simulink model "PubIfDecisionLSM_MDL"  (R2020b)
settings: configuration reference "DspaceConfig" (kept outside this file)
PostLoadFcn:
  | if any(exist('dsrtsu_mdlpostloadfcn', 'file') ~= 0), dsrtsu_mdlpostloadfcn('Execute', bdroot); end
InitFcn:
  | , if any(exist('rtifpga_mdlclblib', 'file') ~= 0), rtifpga_mdlclblib('Init', bdroot); end,
  | , if any(exist('dsmpb_private', 'file') ~= 0), dsmpb_private('dsmpb_mdlclblib', 'Init', bdroot); end,
values from neighbouring files (symbols this model uses):
  P_LSM_ALC_Enable = 0.0    [LSM_Parameter.sldd]
  P_LSM_AwayEdge_offset = 0.1    [LSM_Parameter.sldd]
  P_LSM_CentValidErr = 1.0    [LSM_Parameter.sldd]
  P_LSM_DOP_C0_EN_Limit = 0.8    [LSM_Parameter.sldd]
  P_LSM_DOP_C0_out_Limit = 2.0    [LSM_Parameter.sldd]
  P_LSM_DOP_C1_EN_Limit : value not decoded    [LSM_Parameter.sldd]
  P_LSM_DOP_C1_out_Limit : value not decoded    [LSM_Parameter.sldd]
  P_LSM_DOP_C1AndC2_Lim_X : value not decoded    [LSM_Parameter.sldd]
  P_LSM_DOP_C2_EN_Limit : value not decoded    [LSM_Parameter.sldd]
  P_LSM_DOP_C2_out_Limit : value not decoded    [LSM_Parameter.sldd]
  P_LSM_DOP_In_Pre2Dop_Dis = 1.0    [LSM_Parameter.sldd]
  P_LSM_DOP_Out_Pre2Dop_Dis = 2.0    [LSM_Parameter.sldd]
  P_LSM_DOP_PreDis_X : value not decoded    [LSM_Parameter.sldd]
  P_LSM_DOP_PreDis_Y : value not decoded    [LSM_Parameter.sldd]
  P_LSM_DOPEnableSW = 1.0    [LSM_Parameter.sldd]
  P_LSM_DOPValid_CheckTime = 0.06    [LSM_Parameter.sldd]
  P_LSM_DoubleLine_Curr2Cent_Dislimit = 0.5    [LSM_Parameter.sldd]
  P_LSM_DoubleLine_Dop2Cent_Dislimit = 0.5    [LSM_Parameter.sldd]
  P_LSM_DoubleLine_DOPOut_C1 : value not decoded    [LSM_Parameter.sldd]
  P_LSM_DoubleLine_Pre2Cent_Dislimit = 1.0    [LSM_Parameter.sldd]
  P_LSM_Error_Limit = 0.5    [LSM_Parameter.sldd]
  P_LSM_IFV2CenterAxis = 0.0    [LSM_Parameter.sldd]
  P_LSM_IFV2RearAxis = 0.0    [LSM_Parameter.sldd]
  P_LSM_Line2Edge_limit = 0.5    [LSM_Parameter.sldd]
  P_LSM_Line_Error = 0.1    [LSM_Parameter.sldd]
  P_LSM_LineSTD_Limit = 0.15    [LSM_Parameter.sldd]
  P_LSM_NOH_Switch = 0.0    [LSM_Parameter.sldd]
  P_LSM_OTL_C0_Factor = 1.0    [LSM_Parameter.sldd]
  P_LSM_OTL_C1_Factor = 0.5    [LSM_Parameter.sldd]
  P_LSM_OTL_C2_Factor = 0.5    [LSM_Parameter.sldd]
  P_LSM_Pre2OnlyLineDis = 5.0    [LSM_Parameter.sldd]
  P_LSM_Pre_t = 0.0    [LSM_Parameter.sldd]
  P_LSM_SingleLine_Cent2Edge_Dislimit = 100.0    [LSM_Parameter.sldd]
  P_LSM_SingleLine_Curr2Cent_Dislimit = 0.2    [LSM_Parameter.sldd]
  P_LSM_SingleLine_Dop2Cent_Dislimit = 0.2    [LSM_Parameter.sldd]
  P_LSM_SingleLine_DOPOut_C1 : value not decoded    [LSM_Parameter.sldd]
  P_LSM_SingleLine_Pre2Cent_Dislimit = 0.5    [LSM_Parameter.sldd]
  P_LSM_TJALimitSpd = 60.0    [LSM_Parameter.sldd]
undefined symbols (not defined in the file or in its folder): P_lCS_IFV2CenterAxis, P_LCS_IFV2RearAxis, P_LSM_EntryEdge_offset, P_LSM_EntryLnChngEnSwitch, P_LSM_EntryVanishDis, P_LSM_LinetLostTime, P_LSM_LineWijCal_C12, P_LSM_LineWijCal_C13, P_LSM_MapValid_ErrorSwitch, P_LSM_PosLineLcFac, P_LSM_SpdLim_Stub_Spd, P_LSM_SpdLim_StubLength, P_LSM_SpdTurnAlarm
libraries: simulink x324, TrueDurationTime x11
(part 13 of 25)

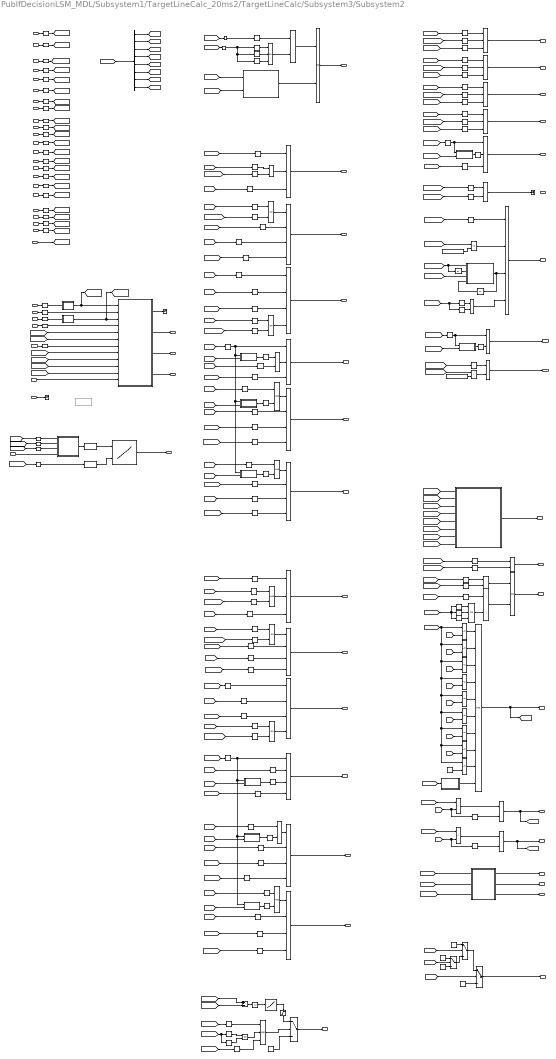
== system PubIfDecisionLSM_MDL/Subsystem1/TargetLineCalc_20ms2/TargetLineCalc/Subsystem3/Subsystem2 ==
  note: 推荐车道
  note: %%未走上汇出线,接管
  note: %%未走上汇出线,接管
  note: 高速或匝道汇出
  note: %%沿着汇出线驶出
  note: en_direction
      | 1 左驶出
      | 2 右驶出
      | 3 左直行
      | 4 右直行
      | 5 驶入
  note: %%未走上汇出线
  note: %%沿着汇出线驶出
  note: %%未走上汇出线
  note: 汇入
  note: 巡航（不存在有效路口）
  note: 左汇出
  note: 汇入或汇出路口有效
  note: 路口限速
  Exit_bIsLineExist : Inport
  f_distance : Inport  Port=2
  b_is_available : Inport  Port=3  OutDataTypeStr=uint8
  i_rec_lanes : Inport  Port=4
  nLaneID : Inport  Port=5
  en_direction : Inport  Port=6  OutDataTypeStr=uint8
  VehInRightmostLane : Inport  Port=7  OutDataTypeStr=boolean
  VehInLeftmostLane : Inport  Port=8  OutDataTypeStr=boolean
  nLaneNum : Inport  Port=9
  i_rec_lanes_num : Inport  Port=10
  " curr_b_vanish_valid" : Inport  Port=11
  " Exit_dDisStart" : Inport  Port=12
  Exit_dC0V : Inport  Port=13
  Entry_bIsLineExist : Inport  Port=14
  Entry_dDisStart : Inport  Port=15
  Entry_dC0V : Inport  Port=16
  " curr_f_vanish_pt_dis " : Inport  Port=17
  rightLane_valid : Inport  Port=18
  rightLane_type : Inport  Port=19
  leftLane_valid : Inport  Port=20
  leftLane_type : Inport  Port=21
  currentLane_type : Inport  Port=22
  VehSpd : Inport  Port=23
  f_end_dis : Inport  Port=24
  PilotRoadSts : Inport  Port=25
  left_b_vanish_valid : Inport  Port=26
  " left_f_vanish_pt_dis" : Inport  Port=27
  right_b_vanish_valid : Inport  Port=28
  right_f_vanish_pt_dis : Inport  Port=29
  currentLane_valid : Inport  Port=30
  HWASts : Inport  Port=31
  1-D Lookup Table : Lookup_n-D  NumberOfTableDimensions=1  BreakpointsForDimension1=P_LSM_SpdLim_StubLength  Table=P_LSM_SpdLim_Stub_Spd  TableDataTypeStr=uint8  ExtrapMethod=Clip  InternalRulePriority=Speed  OutDataTypeStr=uint8  RndMeth=Simplest  InputSameDT=on
  2-D Lookup Table : Lookup_n-D  BreakpointsForDimension1=[0,1,2,3,4,5]  BreakpointsForDimension2=P_LSM_SpdTurnAlarm  Table=reshape([0,1,1,1,1,1,0,0,1,1,1,1,0,0,0,1,1,1,0,0,0,0,1,1,0,0,0,0,0,1,0,0,0,0,0,1],6,6)  TableDataTypeStr=Inherit: Inherit from 'Table data'  InterpMethod=Nearest  InternalRulePriority=Speed  OutDataTypeStr=uint8  RndMeth=Simplest  InputSameDT=on
      settings: InputPortMap=u0,u1
  AND : Logic  AllPortsSameDT=off  OutDataTypeStr=boolean
  AND{1,3..5} (4 alike) : Logic  Operator=OR  AllPortsSameDT=off  OutDataTypeStr=boolean
  AND2 : Logic  AllPortsSameDT=off  OutDataTypeStr=boolean
  Abs : Abs
  Compare To Constant{1,4..5,12,75} (5 alike) : simulink/Logic and Bit Operations/Compare To Constant  relop=<  const=2  OutDataTypeStr=boolean
  Compare To Constant{10,16,46..47,56} (5 alike) : simulink/Logic and Bit Operations/Compare To Constant  relop===  const=5  OutDataTypeStr=boolean
  Compare To Constant11 : simulink/Logic and Bit Operations/Compare To Constant  relop===  const=3  OutDataTypeStr=boolean
  Compare To Constant{13,26,30,65,70,77} (6 alike) : simulink/Logic and Bit Operations/Compare To Constant  relop=<=  const=3  OutDataTypeStr=boolean
  Compare To Constant{14,28,45,48,50,52,61,83,85,95,97} (11 alike) : simulink/Logic and Bit Operations/Compare To Constant  relop===  const=0  OutDataTypeStr=boolean
  Compare To Constant{15,29,40,55,59,62,66,69,72,74,76,82,84,89,91,93} (16 alike) : simulink/Logic and Bit Operations/Compare To Constant  relop=>  const=0  OutDataTypeStr=boolean
  Compare To Constant{17,27,31,67} (4 alike) : simulink/Logic and Bit Operations/Compare To Constant  relop=<  const=1  OutDataTypeStr=boolean
  Compare To Constant{2,9,18..19,21,23..24,32,38,58,60,64,80,90} (14 alike) : simulink/Logic and Bit Operations/Compare To Constant  relop===  const=2  OutDataTypeStr=boolean
  Compare To Constant20 : simulink/Logic and Bit Operations/Compare To Constant  relop=~=  const=5  OutDataTypeStr=boolean
  Compare To Constant{7..8,22,33..35,37,39,51,68,71,81,88,96} (14 alike) : simulink/Logic and Bit Operations/Compare To Constant  relop===  const=1  OutDataTypeStr=boolean
  Compare To Constant25 : simulink/Logic and Bit Operations/Compare To Constant  relop=>  const=3  OutDataTypeStr=boolean
  Compare To Constant3 : simulink/Logic and Bit Operations/Compare To Constant  relop=~=  const=1  OutDataTypeStr=boolean
  Compare To Constant36 : simulink/Logic and Bit Operations/Compare To Constant  relop=~=  const=1  OutDataTypeStr=boolean
  Compare To Constant41 : simulink/Logic and Bit Operations/Compare To Constant  relop=>=  const=50  OutDataTypeStr=boolean
  Compare To Constant42 : simulink/Logic and Bit Operations/Compare To Constant  relop=~=  const=0  OutDataTypeStr=boolean
  Compare To Constant43 : simulink/Logic and Bit Operations/Compare To Constant  relop=~=  const=0  OutDataTypeStr=boolean
  Compare To Constant44 : simulink/Logic and Bit Operations/Compare To Constant  relop=>  const=50  OutDataTypeStr=boolean
  Compare To Constant49 : simulink/Logic and Bit Operations/Compare To Constant  relop===  const=4  OutDataTypeStr=boolean
  Compare To Constant53 : simulink/Logic and Bit Operations/Compare To Constant  relop=<=  const=50  OutDataTypeStr=boolean
  Compare To Constant54 : simulink/Logic and Bit Operations/Compare To Constant  relop=>  const=50  OutDataTypeStr=boolean
  Compare To Constant57 : simulink/Logic and Bit Operations/Compare To Constant  relop=<=  const=50  OutDataTypeStr=boolean
  Compare To Constant6 : simulink/Logic and Bit Operations/Compare To Constant  relop=>  const=3  OutDataTypeStr=boolean
  Compare To Constant63 : simulink/Logic and Bit Operations/Compare To Constant  relop=<  const=50  OutDataTypeStr=boolean
  Compare To Constant73 : simulink/Logic and Bit Operations/Compare To Constant  relop=<  const=50  OutDataTypeStr=boolean
  Compare To Constant78 : simulink/Logic and Bit Operations/Compare To Constant  relop=>=  const=50  OutDataTypeStr=boolean
  Compare To Constant79 : simulink/Logic and Bit Operations/Compare To Constant  relop=<  const=50  OutDataTypeStr=boolean
  Compare To Constant86 : simulink/Logic and Bit Operations/Compare To Constant  relop=>  const=1  OutDataTypeStr=boolean
  Compare To Constant87 : simulink/Logic and Bit Operations/Compare To Constant  relop=>  const=1  OutDataTypeStr=boolean
  Compare To Constant92 : simulink/Logic and Bit Operations/Compare To Constant  relop=~=  const=5  OutDataTypeStr=boolean
  Compare To Constant94 : simulink/Logic and Bit Operations/Compare To Constant  relop=~=  const=6  OutDataTypeStr=boolean
  Constant : Constant  Value=0  OutDataTypeStr=uint8
  Constant1 : Constant  OutDataTypeStr=uint8
  Constant2 : Constant  Value=2  OutDataTypeStr=uint8
  Constant3 : Constant  Value=0  OutDataTypeStr=uint8
  Constant4 : Constant  Value=0  OutDataTypeStr=uint8
  Constant5 : Constant  Value=60  OutDataTypeStr=uint8
  Constant6 : Constant  Value=P_LSM_EntryVanishDis
  Constant7 : Constant  Value=P_LSM_EntryVanishDis
  Data Type Conversion : DataTypeConversion
  Data Type Conversion1 : DataTypeConversion
  Demux : Demux  Outputs=8
  Logical Operator : Logic  Operator=OR  Inputs=3  AllPortsSameDT=off  OutDataTypeStr=boolean
  Logical Operator{1..2,4,8,17,21..22,24,28,31,33,35..37,39} (15 alike) : Logic  AllPortsSameDT=off  OutDataTypeStr=boolean
  Logical Operator{3,6,10,20,25..26,29..30} (8 alike) : Logic  Inputs=3  AllPortsSameDT=off  OutDataTypeStr=boolean
  Logical Operator11 : Logic  Inputs=10  AllPortsSameDT=off  OutDataTypeStr=boolean
  Logical Operator{5,12..13,15,18..19,23,32,34,40} (10 alike) : Logic  Inputs=4  AllPortsSameDT=off  OutDataTypeStr=boolean
  Logical Operator27 : Logic  Operator=OR  AllPortsSameDT=off  OutDataTypeStr=boolean
  Logical Operator38 : Logic  Operator=OR  AllPortsSameDT=off  OutDataTypeStr=boolean
  Logical Operator9 : Logic  Operator=OR  Inputs=3  AllPortsSameDT=off  OutDataTypeStr=boolean
  MATLAB Function : MATLAB Function  TreatAsAtomicUnit=on
  MATLAB Function1 : MATLAB Function  TreatAsAtomicUnit=on
  MATLAB Function2 : MATLAB Function  TreatAsAtomicUnit=on
  MATLAB Function3 : MATLAB Function  TreatAsAtomicUnit=on
  MATLAB Function4 : MATLAB Function  TreatAsAtomicUnit=on
  MATLAB Function5 : MATLAB Function  TreatAsAtomicUnit=on
  OR : Logic  Operator=OR  AllPortsSameDT=off  OutDataTypeStr=boolean
  OR1 : Logic  Inputs=3  AllPortsSameDT=off  OutDataTypeStr=boolean
  Relational Operator : RelationalOperator  Operator=>  OutDataTypeStr=boolean  RndMeth=Simplest
  Relational Operator1 : RelationalOperator  Operator=<=  OutDataTypeStr=boolean  RndMeth=Simplest
  Relational Operator{2..6,10,12..14} (9 alike) : RelationalOperator  Operator=~=  OutDataTypeStr=boolean  RndMeth=Simplest
  Relational Operator7 : RelationalOperator  Operator=>  OutDataTypeStr=boolean  RndMeth=Simplest
  Relational Operator8 : RelationalOperator  Operator=<  OutDataTypeStr=boolean  RndMeth=Simplest
  Saturation : Saturate  UpperLimit=60  LowerLimit=30  OutDataTypeStr=uint8
  Signal Copy{,1..32} (33 alike) : SignalConversion  OverrideOpt=off
  Subsystem : Subsystem
  Subsystem1 : Subsystem
  Subsystem10 : Subsystem
  Subsystem17 : Subsystem
  Subsystem19 : Subsystem
  Subsystem2 : Subsystem  Commented=on
  Subsystem3 : Subsystem
  Subsystem4 : Subsystem
  Subsystem5 : Subsystem
  Subsystem6 : Subsystem
  Subsystem8 : Subsystem
  Subsystem9 : Subsystem
  Subtract : Sum  Inputs=+-
  Switch{,1..3} (4 alike) : Switch  Criteria=u2 > Threshold
  Terminator : Terminator
  Terminator1 : Terminator
  Terminator4 : Terminator
  Unit Delay : UnitDelay  SampleTime=-1  HasFrameUpgradeWarning=on
  Unit Delay1 : UnitDelay  SampleTime=-1  HasFrameUpgradeWarning=on
  StubValid : Outport
  RightStub : Outport  Port=2
  LeftStub : Outport  Port=3
  CruiseValid : Outport  Port=4
  TurnLeft : Outport  Port=5
  TurnRight : Outport  Port=6
  rExitStub1 : Outport  Port=7
  rExitStub2 : Outport  Port=8
  rExitStub3 : Outport  Port=9
  Vanish_turnleft : Outport  Port=10
  EntryStub1 : Outport  Port=11
  CruiseRight : Outport  Port=12
  CruiseLeft : Outport  Port=13
  lExitStub1 : Outport  Port=14
  lExitStub2 : Outport  Port=15
  lExitStub3 : Outport  Port=16
  CruiseTurn : Outport  Port=17
  Forbid_TurnRight : Outport  Port=18
  Forbid_TurnLeft : Outport  Port=19
  OneLane : Outport  Port=20
  EntryStub2 : Outport  Port=21
  EntryStub3 : Outport  Port=22
  EntryStub4 : Outport  Port=23
  EntryStub5 : Outport  Port=24
  EntryStub6 : Outport  Port=25
  EntryStub5_TurnLeft : Outport  Port=26
  rExitStub4_takeover : Outport  Port=27
  lExitStub4_takeover : Outport  Port=28
  EntryStub5_takeover : Outport  Port=29
  Vanish_turnleft_takeover : Outport  Port=30
  turndir : Outport  Port=31
  roadClass : Outport  Port=32
  DecSpd : Outport  Port=33
  ForbidActive : Outport  Port=34
  StudLengthSpd : Outport  Port=35
  EntryStubVanishTurn : Outport  Port=36
  exitTakeOverValid : Outport  Port=37
  wires:
  [VehInLeftmostLane] -> Compare To Constant96/1
  Compare To Constant96/1 -> AND5/2
  Compare To Constant97/1 -> AND5/1
  [CruiseTurn] -> Compare To Constant97/1
  AND5/1 -> Logical Operator19/4
  Compare To Constant71/1 -> AND4/2
  [VehInRightmostLane] -> Compare To Constant71/1
  Compare To Constant95/1 -> AND4/1
  [CruiseTurn] -> Compare To Constant95/1
  AND4/1 -> Logical Operator15/4
  [f_vanish_pt_dis] -> MATLAB Function5/3(f_vanish_pt_dis)
  [b_vanish_valid] -> MATLAB Function5/1(b_vanish_valid), Unit Delay/1
  MATLAB Function5/1(VanishLaneTkOverValid) -> Logical Operator40/3, Unit Delay1/1
  Unit Delay1/1 -> MATLAB Function5/4(VanishLaneTkOverValidK)
  Unit Delay/1 -> MATLAB Function5/2(b_vanish_validK)
  Constant7/1 -> Relational Operator1/2
  Logical Operator4/1 -> Logical Operator40/4  "EntryStub5_takeover"
  Compare To Constant94/1 -> Logical Operator4/2
  Compare To Constant92/1 -> Logical Operator4/1
  [HWASts] -> Compare To Constant92/1, Compare To Constant94/1
  HWASts/1 -> [HWASts]
  Constant6/1 -> Relational Operator/2
  Logical Operator2/1 -> EntryStubVanishTurn/1  "EntryStub5_takeover"
  [f_vanish_pt_dis] -> Relational Operator/1
  Relational Operator/1 -> Logical Operator2/2
  [b_vanish_valid] -> Compare To Constant93/1
  Compare To Constant93/1 -> Logical Operator2/1
  Saturation/1 -> Switch3/1
  Compare To Constant91/1 -> OR1/3
  [f_distance] -> Compare To Constant91/1
  Switch3/1 -> StudLengthSpd/1
  Constant5/1 -> Switch3/3
  1-D Lookup Table/1 -> Saturation/1
  Abs/1 -> 1-D Lookup Table/1
  Subtract/1 -> Abs/1
  OR1/1 -> Switch3/2
  [f_end_dis] -> Subtract/1
  [f_distance] -> Subtract/2
  OR/1 -> OR1/2
  Compare To Constant89/1 -> OR1/1
  Compare To Constant90/1 -> OR/2
  Compare To Constant88/1 -> OR/1
  [b_is_available] -> Compare To Constant89/1
  [en_direction] -> Compare To Constant88/1, Compare To Constant90/1
  Compare To Constant87/1 -> Logical Operator5/4
  [f_distance] -> Compare To Constant87/1
  Compare To Constant86/1 -> Logical Operator12/4
  [f_distance] -> Compare To Constant86/1
  MATLAB Function1/4(ForbidActive) -> ForbidActive/1
  currentLane_valid/1 -> MATLAB Function1/12(currentLane_valid)
  MATLAB Function1/3(DecSpd) -> DecSpd/1
  AND3/1 -> Logical Operator5/1
  [CruiseTurn] -> Compare To Constant85/1
  Compare To Constant85/1 -> AND3/1
  AND2/1 -> Logical Operator20/2
  Compare To Constant84/1 -> AND2/1
  [CruiseTurn] -> Compare To Constant84/1
  AND1/1 -> Logical Operator12/1
  [CruiseTurn] -> Compare To Constant83/1
  Compare To Constant83/1 -> AND1/1
  AND/1 -> Logical Operator3/2
  Compare To Constant82/1 -> AND/1
  [CruiseTurn] -> Compare To Constant82/1
  Data Type Conversion1/1 -> 2-D Lookup Table/2
  Data Type Conversion/1 -> 2-D Lookup Table/1
  2-D Lookup Table/1 -> exitTakeOverValid/1
  MATLAB Function2/1(y) -> Data Type Conversion/1
  [en_direction] -> Signal Copy26/1
  [nLaneID] -> Signal Copy25/1
  [bit1] -> Signal Copy24/1
  [f_distance] -> Signal Copy27/1
  [dDisStart] -> Compare To Constant13/1
  Compare To Constant13/1 -> Logical Operator22/1
  Logical Operator1/1 -> Logical Operator6/2  "rExitStub2"
  [dDisStart] -> Compare To Constant26/1
  Compare To Constant26/1 -> Logical Operator1/2
  MATLAB Function1/2(roadClass) -> roadClass/1
  Signal Copy23/1 -> MATLAB Function1/7(currentLane_type)
  currentLane_type/1 -> Signal Copy23/1
  Signal Copy22/1 -> MATLAB Function1/4(leftLane_type)
  Signal Copy21/1 -> MATLAB Function1/2(rightLane_type)
  leftLane_type/1 -> Signal Copy22/1
  rightLane_type/1 -> Signal Copy21/1
  MATLAB Function1/1(turndir) -> Terminator/1
  Signal Copy20/1 -> Subsystem1/1(In1)
  Signal Copy19/1 -> Subsystem/1(In1)
  [b_vanish_valid] -> MATLAB Function1/5(curr_vanish_valid)
  leftLane_valid/1 -> Signal Copy20/1
  rightLane_valid/1 -> Signal Copy19/1
  Signal Copy2/1 -> [Entry_dDisStart]
  Signal Copy18/1 -> [Entry_dC0V]
  Signal Copy17/1 -> [Entry_bIsLineExist]
  Signal Copy16/1 -> [dDisStart]
  Signal Copy15/1 -> [dC0V]
  Signal Copy14/1 -> [bIsLineExist]
  Signal Copy13/1 -> [en_direction]
  Signal Copy12/1 -> [f_distance]
  Signal Copy11/1 -> [b_is_available]
  Signal Copy10/1 -> [f_vanish_pt_dis]
  Signal Copy9/1 -> [b_vanish_valid]
  Signal Copy8/1 -> [i_rec_lanes_num]
  Signal Copy7/1 -> [nLaneNum]
  Signal Copy6/1 -> [VehInLeftmostLane]
  Signal Copy5/1 -> [VehInRightmostLane]
  Signal Copy4/1 -> [nLaneID]
  Signal Copy3/1 -> [i_rec_lanes]
  Logical Operator/1 -> Logical Operator28/2
  Compare To Constant49/1 -> Logical Operator/3
  Compare To Constant50/1 -> Logical Operator/1
  Compare To Constant11/1 -> Logical Operator/2
  Signal Copy1/1 -> Compare To Constant8/1, Compare To Constant9/1, Compare To Constant10/1  "LSM_en_direction_stub"
  Signal Copy/1 -> Compare To Constant7/1  "LSM_B_IS_Available"
  [bIsLineExist] -> Compare To Constant32/1
  Logical Operator40/1 -> EntryStub5_takeover/1  "EntryStub5_takeover"
  Compare To Constant76/1 -> Logical Operator40/1
  [b_vanish_valid] -> Compare To Constant76/1
  Compare To Constant75/1 -> Logical Operator39/2
  Logical Operator39/1 -> Logical Operator27/1
  [Entry_bIsLineExist] -> Compare To Constant75/1
  Logical Operator38/1 -> StubValid/1  "StubValid"
  Subsystem17/1(enStubExist) -> Logical Operator38/2
  [Entry_bIsLineExist] -> Subsystem17/2(Entry_bIsLineExist)
  [b_is_available] -> Subsystem17/1(b_is_available)
  Logical Operator37/1 -> Vanish_turnleft_takeover/1  "Vanish_turnleft_takeover"
  Compare To Constant74/1 -> Logical Operator37/1  "Vanish_turnleft"
  [b_vanish_valid] -> Compare To Constant74/1
  Compare To Constant73/1 -> Logical Operator37/2  "Vanish_turnleft_takeover"
  [f_vanish_pt_dis] -> Compare To Constant73/1
  Logical Operator36/1 -> Terminator1/1  "EntryStub5_TurnLeft"
  Compare To Constant72/1 -> Logical Operator36/2
  [f_vanish_pt_dis] -> Compare To Constant72/1
  " curr_f_vanish_pt_dis "/1 -> Signal Copy10/1
  Relational Operator1/1 -> Logical Operator40/2
  [f_vanish_pt_dis] -> Relational Operator1/1
  Compare To Constant69/1 -> Logical Operator35/2
  Compare To Constant70/1 -> Logical Operator35/1
  [dDisStart] -> Compare To Constant70/1
  [dC0V] -> Subsystem5/2(u)
  Subsystem5/1(y) -> Compare To Constant69/1
  Compare To Constant68/1 -> Logical Operator34/3
  [en_direction] -> Compare To Constant68/1
  [f_distance] -> Compare To Constant67/1
  Logical Operator34/1 -> lExitStub4_takeover/1  "lExitStub4_takeover"
  Logical Operator35/1 -> Logical Operator34/1
  Compare To Constant67/1 -> Logical Operator34/2
  Subsystem10/1(y) -> Compare To Constant66/1
  [dC0V] -> Subsystem10/2(u)
  [dDisStart] -> Compare To Constant65/1
  Compare To Constant65/1 -> Logical Operator33/1
  Compare To Constant66/1 -> Logical Operator33/2
  Logical Operator33/1 -> Logical Operator32/1
  Logical Operator32/1 -> rExitStub4_takeover/1  "rExitStub4_takeover"
  [f_end_dis] -> Compare To Constant63/1
  [en_direction] -> Compare To Constant64/1
  Compare To Constant64/1 -> Logical Operator32/2
  [b_vanish_valid] -> Compare To Constant62/1
  Compare To Constant62/1 -> Logical Operator36/1
  [Entry_bIsLineExist] -> Compare To Constant60/1
  Compare To Constant60/1 -> Logical Operator31/1, Subsystem8/1(laneValid)
  [Entry_dC0V] -> Subsystem8/2(u)
  Subsystem8/1(y) -> Compare To Constant61/1
  Compare To Constant61/1 -> Logical Operator31/2
  Logical Operator31/1 -> EntryStub6/1  "EntryStub6"
  Logical Operator30/1 -> EntryStub5/1  "EntryStub5"
  Compare To Constant59/1 -> Logical Operator30/2
  Subsystem6/1(y) -> Compare To Constant59/1
  [Entry_dC0V] -> Subsystem6/2(u)
  Compare To Constant58/1 -> Logical Operator30/1, Subsystem6/1(laneValid)
  [Entry_bIsLineExist] -> Compare To Constant58/1
  Logical Operator25/1 -> EntryStub3/1  "EntryStub3"
  [en_direction] -> Compare To Constant47/1  "LSM_Stub_Direction"
  [b_vanish_valid] -> Compare To Constant15/1
  Compare To Constant15/1 -> Logical Operator25/2
  Compare To Constant47/1 -> Logical Operator25/1
  [f_distance] -> Compare To Constant54/1
  Compare To Constant54/1 -> Logical Operator25/3
  Compare To Constant57/1 -> Logical Operator29/3
  [f_distance] -> Compare To Constant57/1
  Compare To Constant56/1 -> Logical Operator29/1
  Compare To Constant55/1 -> Logical Operator29/2
  [b_vanish_valid] -> Compare To Constant55/1
  [en_direction] -> Compare To Constant56/1  "LSM_Stub_Direction"
  Logical Operator29/1 -> EntryStub4/1  "EntryStub4"
  Logical Operator26/1 -> EntryStub2/1  "EntryStub2"
  [en_direction] -> Compare To Constant46/1  "LSM_Stub_Direction"
  [b_vanish_valid] -> Compare To Constant45/1
  Compare To Constant45/1 -> Logical Operator26/2
  Compare To Constant46/1 -> Logical Operator26/1
  [f_distance] -> Compare To Constant53/1
  Compare To Constant53/1 -> Logical Operator26/3
  Compare To Constant44/1 -> Logical Operator10/3
  [f_distance] -> Compare To Constant44/1
  Entry_bIsLineExist/1 -> Signal Copy17/1
  Entry_dDisStart/1 -> Signal Copy2/1
  Entry_dC0V/1 -> Signal Copy18/1
  i_rec_lanes/1 -> Signal Copy3/1
  Demux/2 -> [bit2]
  Demux/3 -> [bit3]
  Demux/1 -> [bit1]
  Demux/8 -> [bit8]
  Demux/7 -> [bit7]
  Demux/6 -> [bit6]
  Demux/4 -> [bit4]
  Demux/5 -> [bit5]
  [i_rec_lanes] -> Demux/1
  Logical Operator24/1 -> [TurnRight], TurnRight/1  "TurnRight"
  Compare To Constant43/1 -> Logical Operator24/2
  Logical Operator21/1 -> [TurnLeft], TurnLeft/1  "TurnLeft"
  Compare To Constant42/1 -> Logical Operator21/2
  Compare To Constant21/1 -> Logical Operator13/3
  Compare To Constant3/1 -> AND/2
  [nLaneID] -> Relational Operator7/1
  Relational Operator5/1 -> Logical Operator11/4
  Relational Operator3/1 -> Logical Operator11/2
  Logical Operator15/1 -> rExitStub1/1  "rExitStub1"
  [en_direction] -> Compare To Constant21/1
  Compare To Constant24/1 -> Logical Operator15/3
  en_direction/1 -> Signal Copy13/1
  [nLaneID] -> Relational Operator3/1, Relational Operator4/1, Relational Operator5/1, Relational Operator10/1, Relational Operator12/1, Relational Operator14/1, Relational Operator13/1, Relational Operator6/1, Relational Operator2/1
  Relational Operator6/1 -> Logical Operator11/5
  [f_distance] -> Compare To Constant17/1
  Compare To Constant16/1 -> Logical Operator10/1
  Compare To Constant2/1 -> Logical Operator3/1
  [bit4] -> Relational Operator5/2
  [en_direction] -> Compare To Constant24/1
  " curr_b_vanish_valid"/1 -> Signal Copy9/1
  Logical Operator13/1 -> rExitStub3/1  "rExitStub3"
  Compare To Constant7/1 -> Logical Operator8/1
  [VehInRightmostLane] -> Compare To Constant3/1
  Exit_dC0V/1 -> Signal Copy15/1
  [bit5] -> Relational Operator6/2
  Compare To Constant14/1 -> Logical Operator10/2
  [bit3] -> Relational Operator4/2
  [bit2] -> Relational Operator3/2
  Compare To Constant25/1 -> Logical Operator15/2
  Logical Operator3/1 -> RightStub/1  "RightStub"
  [dDisStart] -> Compare To Constant25/1
  [b_vanish_valid] -> Compare To Constant14/1
  i_rec_lanes_num/1 -> Signal Copy8/1
  nLaneNum/1 -> Signal Copy7/1
  Logical Operator17/1 -> Logical Operator13/1
  [en_direction] -> Compare To Constant16/1  "LSM_Stub_Direction"
  [bit1] -> Relational Operator7/2, Compare To Constant42/1
  Relational Operator8/1 -> Logical Operator24/1
  [nLaneID] -> Relational Operator8/1
  [bit1] -> Relational Operator8/2, Compare To Constant43/1
  [bit1] -> Relational Operator2/2
  Relational Operator4/1 -> Logical Operator11/3
  Relational Operator2/1 -> Logical Operator11/1
  [en_direction] -> Compare To Constant2/1  "LSM_Stub_Direction"
  f_distance/1 -> Signal Copy12/1
  VehInLeftmostLane/1 -> Signal Copy6/1
  nLaneID/1 -> Signal Copy4/1
  " Exit_dDisStart"/1 -> Signal Copy16/1
  VehInRightmostLane/1 -> Signal Copy5/1
  Compare To Constant17/1 -> Logical Operator13/2
  Logical Operator11/1 -> [CruiseTurn], CruiseTurn/1  "CruiseTurn"
  Logical Operator10/1 -> EntryStub1/1  "EntryStub1"
  [VehInRightmostLane] -> Compare To Constant22/1
  Logical Operator12/1 -> CruiseRight/1  "CruiseRight"
  Compare To Constant22/1 -> AND1/2
  Compare To Constant19/1 -> Logical Operator12/2
  [en_direction] -> Compare To Constant19/1  "LSM_Stub_Direction"
  b_is_available/1 -> Signal Copy11/1
  [b_is_available] -> Signal Copy/1
  [bIsLineExist] -> Compare To Constant1/1
  Compare To Constant1/1 -> Logical Operator3/3
  Exit_bIsLineExist/1 -> Signal Copy14/1
  [bIsLineExist] -> Compare To Constant12/1
  [bIsLineExist] -> Compare To Constant18/1
  Compare To Constant18/1 -> Logical Operator15/1
  Compare To Constant23/1 -> Logical Operator6/1, Subsystem19/1(laneValid), Subsystem9/1(laneValid), Subsystem10/1(laneValid)
  [bIsLineExist] -> Compare To Constant23/1
  Logical Operator6/1 -> rExitStub2/1  "rExitStub2"
  [bIsLineExist] -> Compare To Constant4/1
  Compare To Constant4/1 -> Logical Operator20/3
  [bIsLineExist] -> Compare To Constant5/1
  Compare To Constant36/1 -> AND2/2
  Compare To Constant5/1 -> Logical Operator5/3
  Compare To Constant34/1 -> Logical Operator20/1
  [en_direction] -> Compare To Constant34/1  "LSM_Stub_Direction"
  Compare To Constant33/1 -> Logical Operator5/2
  Compare To Constant35/1 -> AND3/2
  [VehInLeftmostLane] -> Compare To Constant35/1
  [VehInLeftmostLane] -> Compare To Constant36/1
  Logical Operator5/1 -> CruiseLeft/1  "CruiseLeft"
  [en_direction] -> Compare To Constant33/1  "LSM_Stub_Direction"
  Logical Operator20/1 -> LeftStub/1  "LeftStub"
  Logical Operator23/1 -> lExitStub2/1  "lExitStub2"
  [bIsLineExist] -> Compare To Constant38/1
  Compare To Constant38/1 -> Subsystem3/1(laneValid), Subsystem5/1(laneValid), Subsystem4/1(laneValid), Logical Operator23/1
  Compare To Constant32/1 -> Logical Operator19/1
  Compare To Constant31/1 -> Logical Operator18/2
  Logical Operator22/1 -> Logical Operator18/1
  Logical Operator18/1 -> lExitStub3/1  "lExitStub3"
  [en_direction] -> Compare To Constant39/1
  [f_distance] -> Compare To Constant31/1
  Compare To Constant39/1 -> Logical Operator19/3
  [en_direction] -> Compare To Constant37/1
  Logical Operator19/1 -> lExitStub1/1  "lExitStub1"
  Compare To Constant37/1 -> Logical Operator18/3
  Compare To Constant48/1 -> Logical Operator39/1
  [b_is_available] -> Compare To Constant48/1
  Relational Operator10/1 -> Logical Operator11/6
  Relational Operator12/1 -> Logical Operator11/7
  Relational Operator13/1 -> Logical Operator11/8
  [bit6] -> Relational Operator10/2
  [bit7] -> Relational Operator12/2
  [bit8] -> Relational Operator13/2
  Relational Operator7/1 -> Logical Operator21/1
  [en_direction] -> Signal Copy1/1
  Compare To Constant8/1 -> Logical Operator9/1
  Compare To Constant9/1 -> Logical Operator9/2
  Compare To Constant10/1 -> Logical Operator9/3
  Logical Operator9/1 -> Logical Operator8/2
  Logical Operator8/1 -> Logical Operator38/1  "LSM_B_StubValid"
  Compare To Constant12/1 -> Logical Operator12/3
  Relational Operator14/1 -> Logical Operator11/9
  Constant/1 -> Relational Operator14/2
  Logical Operator28/1 -> Logical Operator27/2
  [en_direction] -> Compare To Constant49/1, Compare To Constant11/1, Compare To Constant50/1
  [b_is_available] -> Compare To Constant51/1
  Compare To Constant51/1 -> Logical Operator28/1
  Logical Operator27/1 -> CruiseValid/1  "CruiseValid"
  [i_rec_lanes] -> MATLAB Function/2(i_rec_lanes)
  [nLaneID] -> MATLAB Function/1(nLaneID)
  MATLAB Function/1(Forbid_TurnRight) -> Forbid_TurnRight/1
  MATLAB Function/2(Forbid_TurnLeft) -> Forbid_TurnLeft/1
  MATLAB Function/3(OneLane) -> OneLane/1
  [i_rec_lanes_num] -> MATLAB Function/3(i_rec_lanes_num)
  Subsystem19/1(y) -> Compare To Constant52/1
  [dC0V] -> Subsystem19/2(u)
  Compare To Constant52/1 -> Logical Operator1/1
  Compare To Constant29/1 -> Logical Operator17/2
  Compare To Constant77/1 -> Logical Operator17/1
  [dDisStart] -> Compare To Constant77/1
  [dC0V] -> Subsystem9/2(u)
  Subsystem9/1(y) -> Compare To Constant29/1
  [dDisStart] -> Compare To Constant6/1
  Compare To Constant6/1 -> Logical Operator19/2
  Compare To Constant28/1 -> Logical Operator23/3
  Compare To Constant30/1 -> Logical Operator23/2
  [dDisStart] -> Compare To Constant30/1
  [dC0V] -> Subsystem4/2(u)
  Subsystem4/1(y) -> Compare To Constant28/1
  Subsystem3/1(y) -> Compare To Constant40/1
  [dC0V] -> Subsystem3/2(u)
  Compare To Constant40/1 -> Logical Operator22/2
  [i_rec_lanes] -> MATLAB Function3/1(i_rec_lanes)
  MATLAB Function3/1(y) -> Logical Operator11/10
  Signal Copy24/1 -> MATLAB Function2/1(nLaneNum)  "LSM_nLaneNum"
  Signal Copy25/1 -> MATLAB Function2/2(nLaneID)  "LSM_nLaneID"
  Signal Copy26/1 -> MATLAB Function2/3(en_direction)
  Signal Copy27/1 -> Data Type Conversion1/1  "LSM_f_distance"
  f_end_dis/1 -> Signal Copy28/1
  Signal Copy28/1 -> [f_end_dis]
  [f_distance] -> Compare To Constant27/1
  Compare To Constant27/1 -> Logical Operator32/3
  [f_end_dis] -> Compare To Constant41/1
  Compare To Constant41/1 -> Logical Operator13/4
  [f_end_dis] -> Compare To Constant78/1
  Compare To Constant78/1 -> Logical Operator18/4
  [f_end_dis] -> Compare To Constant79/1
  Compare To Constant79/1 -> Logical Operator34/4
  Subsystem/1(y) -> MATLAB Function1/1(rightLane_valid), [rightLane_valid]
  Subsystem1/1(y) -> MATLAB Function1/3(leftLane_valid), [leftLane_valid]
  VehSpd/1 -> Terminator4/1
  PilotRoadSts/1 -> MATLAB Function2/4(PilotRoadSts)
  left_b_vanish_valid/1 -> Signal Copy30/1
  " left_f_vanish_pt_dis"/1 -> Signal Copy29/1
  Signal Copy30/1 -> [left_b_vanish_valid]
  Signal Copy29/1 -> [left_f_vanish_pt_dis]
  Signal Copy31/1 -> [right_f_vanish_pt_dis]
  Signal Copy32/1 -> [right_b_vanish_valid]
  right_f_vanish_pt_dis/1 -> Signal Copy31/1
  right_b_vanish_valid/1 -> Signal Copy32/1
  [f_vanish_pt_dis] -> MATLAB Function1/6(curr_vanish_pt_dis)
  [left_b_vanish_valid] -> MATLAB Function1/8(left_vanish_valid)
  [left_f_vanish_pt_dis] -> MATLAB Function1/9(left_vanish_pt_dis)
  [right_b_vanish_valid] -> MATLAB Function1/10(right_vanish_valid)
  [right_f_vanish_pt_dis] -> MATLAB Function1/11(right_vanish_pt_dis)
  MATLAB Function4/1(y) -> Vanish_turnleft/1
  [b_vanish_valid] -> MATLAB Function4/3(curr_vanish_valid)
  [f_vanish_pt_dis] -> MATLAB Function4/4(curr_vanish_pt_dis)
  [right_f_vanish_pt_dis] -> MATLAB Function4/8(right_vanish_pt_dis)
  [right_b_vanish_valid] -> MATLAB Function4/7(right_vanish_valid)
  [left_f_vanish_pt_dis] -> MATLAB Function4/6(left_vanish_pt_dis)
  [left_b_vanish_valid] -> MATLAB Function4/5(left_vanish_valid)
  [leftLane_valid] -> MATLAB Function4/2(leftLane_valid)
  [rightLane_valid] -> MATLAB Function4/1(rightLane_valid)
  Compare To Constant63/1 -> Logical Operator32/4
  [CruiseTurn] -> Switch/2
  Switch/1 -> turndir/1
  [TurnLeft] -> Switch1/2
  Constant1/1 -> Switch1/1
  [TurnRight] -> Switch2/2
  Constant2/1 -> Switch2/1
  Switch2/1 -> Switch1/3
  Switch1/1 -> Switch/1
  Constant3/1 -> Switch2/3
  Constant4/1 -> Switch/3
  Compare To Constant20/1 -> Logical Operator30/3
  [en_direction] -> Compare To Constant20/1  "LSM_Stub_Direction"
  [en_direction] -> Compare To Constant80/1
  Compare To Constant80/1 -> Logical Operator6/3
  Compare To Constant81/1 -> Logical Operator23/4
  [en_direction] -> Compare To Constant81/1

== system PubIfDecisionLSM_MDL/Subsystem1/TargetLineCalc_20ms2/TargetLineCalc/Subsystem3/Subsystem3 ==
  PilotTurnSwSts : Inport
  nLaneID : Inport  Port=2
  Compare To Constant2 : simulink/Logic and Bit Operations/Compare To Constant  relop===  const=1  OutDataTypeStr=boolean
  Compare To Constant3 : simulink/Logic and Bit Operations/Compare To Constant  relop===  const=2  OutDataTypeStr=boolean
  Constant : Constant  OutDataTypeStr=uint8
  Constant1 : Constant  Value=2  OutDataTypeStr=uint8
  Constant2 : Constant  Value=0  OutDataTypeStr=uint8
  Logical Operator1 : Logic  AllPortsSameDT=off  OutDataTypeStr=boolean
  Logical Operator2 : Logic  AllPortsSameDT=off  OutDataTypeStr=boolean
  Relational Operator1 : RelationalOperator  Operator=<  OutDataTypeStr=boolean  RndMeth=Simplest
  Relational Operator2 : RelationalOperator  Operator=>  OutDataTypeStr=boolean  RndMeth=Simplest
  Switch : Switch  Criteria=u2 > Threshold
  Switch1 : Switch  Criteria=u2 > Threshold
  Unit Delay{,1..3} (4 alike) : UnitDelay  SampleTime=-1  HasFrameUpgradeWarning=on
  LaneChange : Outport
  wires:
  Switch/1 -> LaneChange/1  "LaneChange"
  Relational Operator2/1 -> Logical Operator2/2
  nLaneID/1 -> Relational Operator1/1, Unit Delay/1, Unit Delay1/1, Relational Operator2/1
  Switch1/1 -> Switch/3
  Compare To Constant3/1 -> Logical Operator2/1
  Unit Delay1/1 -> Relational Operator2/2
  Constant1/1 -> Switch1/1
  Unit Delay3/1 -> Compare To Constant2/1
  Logical Operator2/1 -> Switch1/2
  PilotTurnSwSts/1 -> Unit Delay3/1, Unit Delay2/1
  Unit Delay/1 -> Relational Operator1/2
  Logical Operator1/1 -> Switch/2
  Unit Delay2/1 -> Compare To Constant3/1
  Constant2/1 -> Switch1/3
  Constant/1 -> Switch/1
  Compare To Constant2/1 -> Logical Operator1/1
  Relational Operator1/1 -> Logical Operator1/2

== system PubIfDecisionLSM_MDL/Subsystem1/TargetLineCalc_20ms2/TargetLineCalc/Subsystem3/Subsystem4 ==
  PilotRoadSts : Inport
  en_direction : Inport  Port=2
  f_vanish_pt_dis : Inport  Port=3
  changeVoice : Inport  Port=4
  b_vanish_valid : Inport  Port=5
  exitTakeOverValid : Inport  Port=6
  lExitStub4_takeover : Inport  Port=7
  rExitStub4_takeover : Inport  Port=8
  f_distance : Inport  Port=9
  Double_Line_Lost : Inport  Port=10
  LaneNum : Inport  Port=11
  NoPUCR : Inport  Port=12
  NoPUCR_Dis : Inport  Port=13
  HWASts : Inport  Port=14
  Chart : Stateflow chart  TreatAsAtomicUnit=on
      settings: PortSchema="{\"entries\":[{\"content\":{\"sides\":[{\"content\":{\"connectorIds\":[\"In1\",\"In7\",\"In2\",\"In3\",\"In4\",\"In5\",\"In6\",\"In8\",\"In9\",\"In10\",\"In11\",\"In12\",\"In13\",\"In14\",\"In15\"]},\"type\":\"ConnectorPlacement.EquallySpacedRectSide\",\"uuid\":\"ffbd8463-567a-4659-b8b5-1d92828b502e\"},{\"content\":{\"connectorIds\":[\"Out1\"],\"side\":\"RIGHT\"},\"type\":\"ConnectorPlacement.EquallySpacedRectSide\",\"uuid\":\"a8d4ede4-058c-411e-a1bb-a05fa58933cd\"},{\"content\":{\"connectorIds\":[],\"side\":\"TOP\"},\"type\":\"ConnectorPlacement.EquallySpacedRectSide\",\"uuid\":\"cb34091e-f6c1-4e39-8b68-2bb4c65a08b7\"},{\"content\":{\"connectorIds\":[],\"side\":\"HIDDEN\"},\"type\":\"ConnectorPlacement.EquallySpacedRectSide\",\"uuid\":\"3139b7f1-1c79-4b06-a78a-de5284464f98\"}]},\"type\":\"ConnectorPlacement.EquallySpacedConnector\",\"uuid\":\"8437a6c5-b71e-48c0-980a-51389f42da06\"}],\"packageUris\":[\"http://schema.mathworks.com/mf0/Connector/R2020b\"],\"version\":\"1.0\"}"
  Compare To Constant1 : simulink/Logic and Bit Operations/Compare To Constant  relop=>  const=0  OutDataTypeStr=boolean
  Compare To Constant67 : simulink/Logic and Bit Operations/Compare To Constant  relop=>  const=0  OutDataTypeStr=boolean
  Constant : Constant  Value=P_LSM_EntryVanishDis
  OR : Logic  Operator=OR  AllPortsSameDT=off  OutDataTypeStr=boolean
  Signal Copy{5..6,8,10..12} (6 alike) : SignalConversion  OverrideOpt=off
  Unit Delay1 : UnitDelay  SampleTime=-1  HasFrameUpgradeWarning=on
  NOH_HMI_Voice : Outport
  wires:
  HWASts/1 -> Chart/15(HWASts)
  LaneNum/1 -> Chart/11(LaneNum)
  f_distance/1 -> Chart/9(f_distance)
  Double_Line_Lost/1 -> Chart/10(Double_Line_Lost)
  PilotRoadSts/1 -> Signal Copy5/1
  en_direction/1 -> Signal Copy8/1
  f_vanish_pt_dis/1 -> Signal Copy10/1
  exitTakeOverValid/1 -> Signal Copy6/1
  Chart/1(NOH_HMI_Voice) -> NOH_HMI_Voice/1
  NoPUCR_Dis/1 -> Chart/13(NoPUCR_Dis)
  NoPUCR/1 -> Chart/12(NoPUCR)
  b_vanish_valid/1 -> Signal Copy12/1
  Signal Copy6/1 -> Chart/6(exitTakeOverValid)  "LSM_exitTakeOverValid"
  lExitStub4_takeover/1 -> Compare To Constant67/1
  Constant/1 -> Chart/14(EnVanDis)
  Signal Copy12/1 -> Chart/5(b_vanish_valid)
  Unit Delay1/1 -> Chart/7(PilotRoadStsK)
  Signal Copy10/1 -> Chart/3(f_vanish_pt_dis)
  Compare To Constant1/1 -> OR/2
  rExitStub4_takeover/1 -> Compare To Constant1/1
  changeVoice/1 -> Signal Copy11/1
  OR/1 -> Chart/8(ExitStub4_takeover)
  Compare To Constant67/1 -> OR/1
  Signal Copy11/1 -> Chart/4(changeVoice)
  Signal Copy8/1 -> Chart/2(en_direction)  "LSM_EN_Direction"
  Signal Copy5/1 -> Chart/1(PilotRoadSts), Unit Delay1/1

== system PubIfDecisionLSM_MDL/Subsystem1/TargetLineCalc_20ms/TargetLineCalc/Subsystem3/Subsystem2/Subsystem ==
  u : Inport
  MATLAB Function14 : MATLAB Function  TreatAsAtomicUnit=on
  Unit Delay : UnitDelay  SampleTime=-1  HasFrameUpgradeWarning=on
  y : Outport
  wires:
  MATLAB Function14/1(y) -> y/1
  Unit Delay/1 -> MATLAB Function14/2(i_k)
  u/1 -> MATLAB Function14/1(u)
  MATLAB Function14/2(i) -> Unit Delay/1

== system PubIfDecisionLSM_MDL/Subsystem1/TargetLineCalc_20ms/TargetLineCalc/Subsystem3/Subsystem2/Subsystem1 ==
  u : Inport
  MATLAB Function14 : MATLAB Function  TreatAsAtomicUnit=on
  Unit Delay : UnitDelay  SampleTime=-1  HasFrameUpgradeWarning=on
  y : Outport
  wires:
  MATLAB Function14/2(i) -> Unit Delay/1
  u/1 -> MATLAB Function14/1(u)
  Unit Delay/1 -> MATLAB Function14/2(i_k)
  MATLAB Function14/1(y) -> y/1
